simulink model "rtwdemo_forsl"  (Simulink 7.1)
settings: Solver=FixedStepDiscrete  StartTime=0.0  StopTime=10.0  FixedStep=.01  RelTol=1e-3
settings Model: Creator=ajayaram  LastModifiedBy=ajayaram
settings SolverCC: AutoInsertRateTranBlk=on
settings DataIOCC: SaveOutput=off  SaveTime=off
settings OptimizationCC: InlineParams=on  InlineInvariantSignals=on  EnforceIntegerDowncast=off  StateBitsets=on  DataBitsets=on  UseTempVars=on  OptimizeModelRefInitCode=on  LifeSpan=1
settings DebuggingCC: SaveWithParameterizedLinksMsg=none
settings RTWCC: SystemTargetFile=ert.tlc  GenCodeOnly=on  GenerateMakefile=off  TemplateMakefile=ert_default_tmf  Description=Real-Time Workshop Embedded Coder (no auto configuration)  GenerateReport=on  RTWVerbose=off  ProcessScript=ert_make_rtw_hook  IncludeHyperlinkInReport=on  LaunchReport=on
settings CodeAppCC: GenerateComments=off  IgnoreCustomStorageClasses=off  CustomSymbolStrGlobalVar=rt$N$M  CustomSymbolStrType=$N$M  CustomSymbolStrFcn=$N$M$F  CustomSymbolStrMacro=$N$M  SimulinkBlockComments=off
settings ERTTargetCC: SuppressErrorStatus=on  SupportAbsoluteTime=off  SupportNonFinite=off  SupportComplex=off  InlinedParameterPlacement=NonHierarchical  RootIOFormat=Structure reference  ERTCustomFileTemplate=example_file_process.tlc

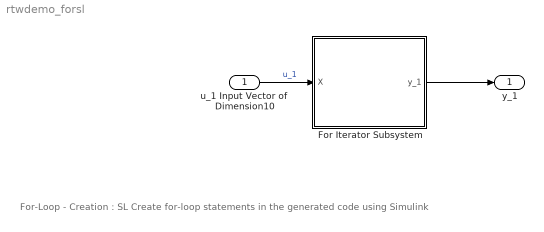
== system rtwdemo_forsl ==
  note: For-Loop - Creation : SL
      | Create for-loop statements in the
      | generated code using Simulink
  "u_1 Input Vector of  Dimension10 " : Inport  PortDimensions=10  OutDataType=sfix(16)  OutScaling=2^0
  For Iterator Subsystem : Subsystem  TreatAsAtomicUnit=on
  y_1 : Outport  OutDataType=sfix(16)  OutScaling=2^0
  wires:
  "u_1 Input Vector of  Dimension10 "/1 -> For Iterator Subsystem/1(X)  "u_1"
  For Iterator Subsystem/1(y_1) -> y_1/1

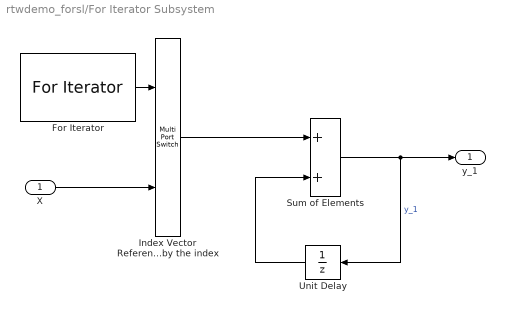
== system rtwdemo_forsl/For Iterator Subsystem ==
  X : Inport  OutDataType=sfix(16)  OutScaling=2^0
  For Iterator : ForIterator  ResetStates=reset  IterationLimit=10  IndexMode=Zero-based
  Index Vector References the element specified by the index : MultiPortSwitch  Inputs=1  zeroidx=on
  Sum of Elements : Sum  OutDataType=sfix(16)  OutScaling=2^-10
  Unit Delay : UnitDelay  Orientation=left  SampleTime=-1  StateIdentifier=x_1
      settings: RTWStateStorageClass=ExportedGlobal
  y_1 : Outport  OutDataType=sfix(16)  OutScaling=2^0
  wires:
  For Iterator/1 -> Index Vector References the element specified by the index/1
  X/1 -> Index Vector References the element specified by the index/2
  Index Vector References the element specified by the index/1 -> Sum of Elements/1
  Sum of Elements/1 -> y_1/1, Unit Delay/1  "y_1"
  Unit Delay/1 -> Sum of Elements/2
